simulink model "43_BusNetworkElectricityTransmissionModel"  (R2023b)
settings: Solver=VariableStepAuto  StartTime=0.0  StopTime=0.8  RelTol=1e-3
model workspace (MAT data in the model file):
  BESS_Fp_KDroop = 0.025
  BESS_KSI = 817
  BESS_PWM_fs = 560
  BESS_P_Ki = 0.5
  BESS_P_Kp = 0.0636
  BESS_Pnom = 3000000
  BESS_Q_Ki = 1
  BESS_Q_Kp = 0.0257
  BESS_Vd_Ki = 850
  BESS_Vd_Kp = 0.216
  BESS_Vnom = 1000
  BESS_Vq_KDroop = 0.025
  BESS_Vq_Ki = 850
  BESS_Vq_Kp = 0.216
  Compensation_Ki = 30
  Compensation_Kp = 3
  DC_Ki = 400
  DC_Kp = 8
  F = 0.01
  Flux_min = 0.5
  Grid_Freq_PWM = 2700
  Grid_Ireg_Ki = 5
  Grid_Ireg_Kp = 0.83
  Grid_Ireg_lim = 1.1
  Grid_Modindex_Upper = 1.1
  Grid_conv_Imax = 0.8
  H = 0.685
  Idref_max = 0.9
  Iqref_Tc = 0.3
  Ki_Var = 0.05
  Ki_Vreg = 20
  Ksh = 1.1
  L_pu = 0.3
  Llr = 0.16
  Lls = 0.18
  Lm = 2.9
  LowLoad_P = 130
  Nb_wt = 6
  P_mech = 1080000
  PeakShav_P = 200
  Pitch_Ki = 0
  Pitch_Kp = 150
  Pitch_Max = 27
  Pitch_Tc = 0.01
  Pitch_rate = 10
  Q_Filt = 50
  R_pu = 0.003
  Rotor_Freq_PWM = 1620
  Rotor_Ireg_Ki = 8
  Rotor_Ireg_Kp = 0.6
  Rotor_Ireg_lim = 0.1
  Rotor_Modindex_Upper = 2
  Rr = 0.016
  Rs = 0.023
  SOCBESS : Simulink.Parameter (value not decoded)
  T_set = 0.0001
  Tp = 5e-05
  Ts = 5e-06
  Var_C_Filt = 720000
  Var_reg_max = 1.1
  Var_reg_min = 0.9
  WT_Coeff = [0.645 116 0.4 5 21 0.00912 0.08 0.035]
  WT_H = 4.32
  WT_IGBTRon = 5.931
  WT_Param = [91.204 10143]
  Wind_Freq_Filt = 10000
  Wind_Freq_nom = 60
  Wind_P_nom = 1200000
  Wind_Rotor_V_nom = 1950
  Wind_V_nom = 500
  Zeta_Filt = 0.707106781187
  init = [-0.2 0 0 0 0 0 0 0]
  p = 3
  torque0 = 0.83
  v_Ki = 0.1
  v_Kp = 3.6
  v_Max = 1.2
  v_Min = 0.7
  v_T = 5
  vreg_max = 1
  wind_VDC_nom = 1150
  wt0 = 1.2
undefined symbols (not defined in the file): D1, D11, Delta, DiscIntNeverNeededParam, Iabc, Ion, Lithium, P, Q, Vabc
libraries: powerlib_extras x156, spsSeriesRLCBranchLib x66, spsLoadFlowBusLib x43, spsThreePhaseSeriesRLCLoadLib x33, spsThreePhaseTransformerTwoWindingsLib x32, spsThreePhaseVIMeasurementLib x30, simulink_extras x30, spsDistributedParametersLineLib x22, spsGenericPowerSystemStabilizerLib x20, spsSynchronousMachinepuStandardLib x10, spsExcitationSystemLib x10, spsHydraulicTurbineandGovernorLib x10
(part 4 of 19)

== system 43_BusNetworkElectricityTransmissionModel/PSS_Equation ==
  In1 : Inport
  1 : Constant
  Sum : Sum  Inputs=|++
  wires:
  In1/1 -> Sum/1
  1/1 -> Sum/2
  Sum/1 -> [PSS_modes]

== system 43_BusNetworkElectricityTransmissionModel/Regulators 10 ==
  m : Inport
  Bus Selector : BusSelector  OutputSignals="dq0 components.Stator voltage  vq (pu),dq0 components.Stator voltage  vd (pu),Mechanical.Rotor speed  wm  (pu),Output active power   Peo (pu)"
  Constant : Constant  Value=0.81818
  Constant1 : Constant
  Math Function : Math  Operator=hypot
  Turbine and Excitation Regulators : Subsystem
  Pm : Outport
  Vf : Outport  Port=2
  tag scope: Vm10=global, w10=global
  wires:
  Bus Selector/4 -> Turbine and Excitation Regulators/3(Pe 0)  "<Output active power   Peo (pu)>"
  Constant1/1 -> Turbine and Excitation Regulators/4(Vref)
  Bus Selector/3 -> [w10], Turbine and Excitation Regulators/2(w)  "<Rotor speed  wm  (pu)>"
  Turbine and Excitation Regulators/1(Pm) -> Pm/1
  m/1 -> Bus Selector/1
  Turbine and Excitation Regulators/2(Vf) -> Vf/1
  Bus Selector/2 -> Math Function/1  "<Stator voltage  vd (pu)>"
  Math Function/1 -> [Vm10], Turbine and Excitation Regulators/5(Vm)
  Bus Selector/1 -> Math Function/2  "<Stator voltage  vq (pu)>"
  Constant/1 -> Turbine and Excitation Regulators/1(pref)
